simulink model "wind_turbine_modelling"  (R2018a)
settings: Solver=VariableStepAuto  StartTime=0.0  StopTime=10.0  RelTol=1e-3
libraries: powerlib x5, re_lib x1
settings Model: Creator=vardh  LastModifiedBy=vardh

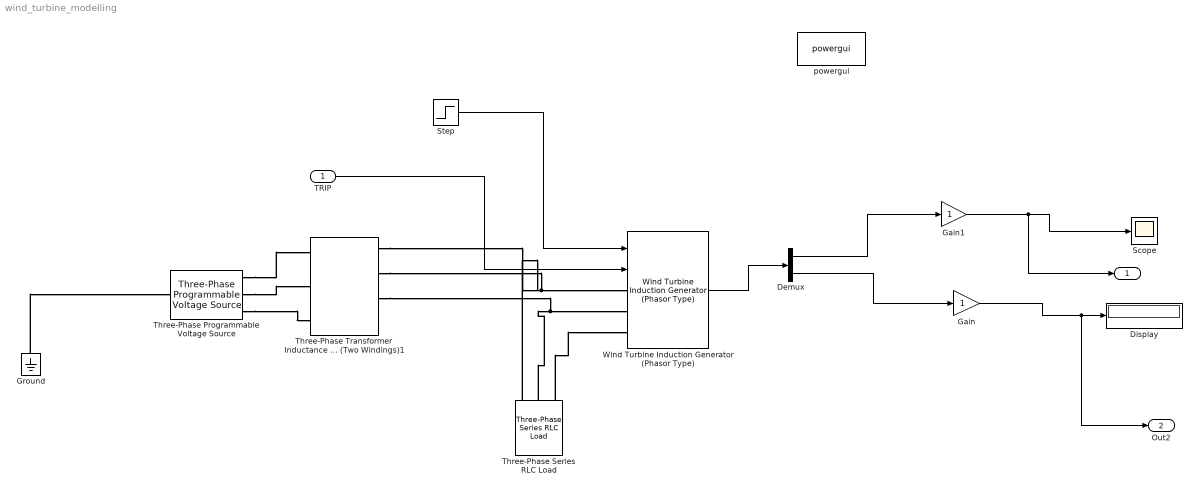
== system wind_turbine_modelling ==
  TRIP : Inport
  Demux : Demux  Outputs=2
  Display : Display
  Gain : Gain
  Gain1 : Gain
  Ground : powerlib/Elements/Ground  LConnTagsString=a
  Scope : Scope
  Step : Step  Time=10  After=10  SampleTime=0
  Three-Phase Programmable Voltage Source : powerlib/Electrical Sources/Three-Phase Programmable Voltage Source  PositiveSequence="[25000  0 60]"  VariationEntity=None  VariationType=Table of time-amplitude pairs  VariationTypeAlt=Step  VariationStep=0.5  VariationRate=10  VariationMagnitude=0.3  VariationFrequency=2  VariationTiming=[1 2]  VariationPhaseA=off  Amplitudes=[1 0.8 1.2 1.0]  TimeValues=[0 0.1 0.15 0.2]  HarmonicGeneration=off  HarmonicA=[3 0.2 -25 0]  HarmonicB=[2 0.15 35 2]  Timing="[0.05  3]"  BusType=swing  Pref=0  Qref=0  Qmin=-inf  Qmax=inf
  Three-Phase Series RLC Load : powerlib/Elements/Three-Phase Series RLC Load  LConnTagsString=A|B|C  RConnTagsString=N  Configuration=Y (neutral)  NominalVoltage=1000  Vabc=[1e3 1e3 1e3]  Vabcp=[1e3 1e3 1e3]  NominalFrequency=60  UnbalancedPower=off  ActivePower=0  InductivePower=0  CapacitivePower=400e3  Pabc=[10e3 9e3 11e3]  QLabc=[100 90 110]  QCabc=[100 90 110]  Pabcp=[10e3 9e3 11e3]  QLabcp=[100 90 110]  QCabcp=[100 90 110]  Measurements=None  LoadType=constant Z
  Three-Phase Transformer Inductance Matrix Type (Two Windings)1 : powerlib/Elements/Three-Phase Transformer Inductance Matrix Type (Two Windings)  CoreType=Three-limb or five-limb core  Winding1Connection=Yg  Winding2Connection=Yn  AutoTransformer=off  Measurements=None  NominalPower=[400e6, 60]  VLLnom=[25000,575]  WindingResistances=[0.01, 0.01]  NoLoadIexcPos=2  NoLoadPlossPos=10000  ShortCircuitReactancePos=0.06  ShortCircuitReactancePosAuto=0.06  NoLoadIexcZero=100  NoLoadPlossZero=1500  ShortCircuitReactanceZero=0.03  ShortCircuitReactanceZeroAuto=0.03
      settings: SourceProductName=Simscape Power Systems  SourceProductBaseCode=PS
  Wind Turbine Induction Generator (Phasor Type) : re_lib/Wind Generation/Wind Turbine Induction Generator (Phasor Type)  ExternalTm=off  nom=[1.5e6/0.9, 575, 60]  sta=[ 0.004843, 0.1248]  rot=[ 0.004377, 0.1791]  Lm=6.77  mec=[5.04, 0.01, 3]  init="[ -0.01,0,   0,0,0,   0,0,0 ]"  pitch_angle=10  Pmec=1.5e6  wind_base=12  speed_nom=1  P_wind_base=1  K_pitch_gain=[5 25]  pitch_max=45  pitch_rate=2
      settings: SourceProductName=Simscape Power Systems  SourceProductBaseCode=PS
  powergui : powerlib/powergui  Priority=1  SimulationMode=Phasor  SampleTime=50e-6  frequency=60  Iterations=50  frequencyindice=60  Pbase=100e6  ErrMax=1e-4  UnitsV=kV  UnitsW=MW  buscounter=0  FunctionMessages=off  echomessages=off  EnableUseOfTLC=off  CurrentSourceSwitches=off  DisableSnubberDevices=off  DisableRonSwitches=off  DisableVfSwitches=off  DisplayEquations=off  SolverType=Tustin/Backward Euler (TBE)  Interpol=off  ExternalGateDelay=off  methode=off  Ts=100  x0status=blocks  SPID=on  SwTol=0  HookPort=off  RestoreLinks=warning  ResistiveCurrentMeasurement=off  Frange=[0:2:500]  Ylog=off  Xlog=on  ShowGrid=off  save=off  variable=ZData  structure=0  ZoomFFT=off  StartTime=0.0  cycles=1  DisplayStyle=1  fundamental=60  FreqAxis=off  MaxFrequency=1000  frequencyindicesteady=1  RmsSteady=1  display=off
  " " : Outport  SignalName=P Out
  Out2 : Outport  Port=2  SignalName=Q Out
  wires:
  Step/1 -> Wind Turbine Induction Generator (Phasor Type)/1
  Wind Turbine Induction Generator (Phasor Type)/1 -> Demux/1
  Demux/1 -> Gain1/1
  Demux/2 -> Gain/1
  Gain1/1 -> " "/1, Scope/1
  Gain/1 -> Out2/1, Display/1
  TRIP/1 -> Wind Turbine Induction Generator (Phasor Type)/2
  connections:
  Three-Phase Programmable Voltage Source/RConn1 -- Three-Phase Transformer Inductance Matrix Type (Two Windings)1/LConn1
  Three-Phase Programmable Voltage Source/RConn2 -- Three-Phase Transformer Inductance Matrix Type (Two Windings)1/LConn2
  Three-Phase Programmable Voltage Source/RConn3 -- Three-Phase Transformer Inductance Matrix Type (Two Windings)1/LConn3
  Three-Phase Transformer Inductance Matrix Type (Two Windings)1/RConn1 -- Three-Phase Series RLC Load/LConn1 -- Three-Phase Transformer Inductance Matrix Type (Two Windings)1/RConn2 -- Wind Turbine Induction Generator (Phasor Type)/LConn1
  Three-Phase Series RLC Load/LConn2 -- Three-Phase Transformer Inductance Matrix Type (Two Windings)1/RConn3 -- Wind Turbine Induction Generator (Phasor Type)/LConn2
  Three-Phase Series RLC Load/LConn3 -- Wind Turbine Induction Generator (Phasor Type)/LConn3
  Ground/LConn1 -- Three-Phase Programmable Voltage Source/LConn1
